simulink library "AeroSim"  (Simulink 7.8)
settings: Solver=ode45  StartTime=0.0  StopTime=10.0  RelTol=1e-3
libraries: AeroSim x3
settings Model: Creator=Ryan  LastModifiedBy=Ryan

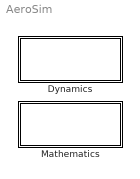
== system AeroSim ==
  Dynamics : Subsystem
      mask Display: disp('Dynamics')
  Mathematics : Subsystem
      mask Display: disp('Mathematics')

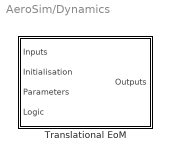
== system AeroSim/Dynamics ==
  Translational EoM : Subsystem

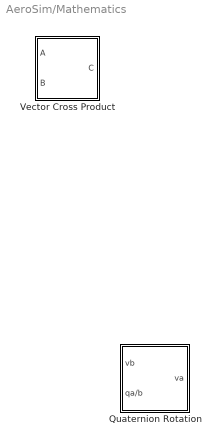
== system AeroSim/Mathematics ==
  Quaternion Rotation : Subsystem
  Vector Cross Product : Subsystem

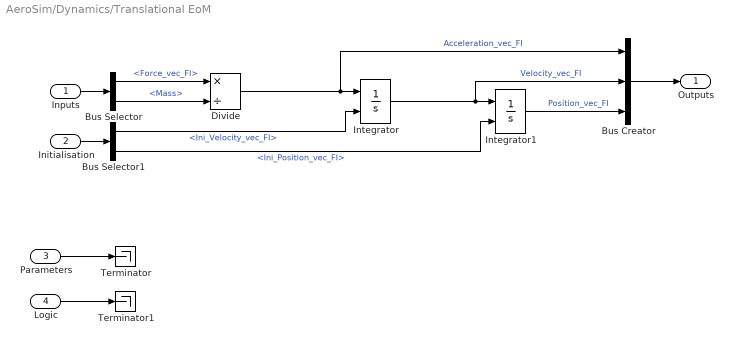
== system AeroSim/Dynamics/Translational EoM ==
  Inputs : Inport  OutDataTypeStr=Bus: Dynamics_TranslationalEoM_Inputs
  Initialisation : Inport  Port=2  OutDataTypeStr=Bus: Dynamics_TranslationalEoM_Initialisation
  Parameters : Inport  Port=3
  Logic : Inport  Port=4
  Bus Creator : BusCreator  Inputs=3
  Bus Selector : BusSelector  OutputSignals=Force_vec_FI,Mass
  Bus Selector1 : BusSelector  OutputSignals=Ini_Velocity_vec_FI,Ini_Position_vec_FI
  Divide : Product  Inputs=*/
  Integrator : Integrator  InitialConditionSource=external
  Integrator1 : Integrator  InitialConditionSource=external
  Terminator : Terminator
  Terminator1 : Terminator
  Outputs : Outport  OutDataTypeStr=Bus: Dynamics_TranslationalEoM_Outputs
  wires:
  Parameters/1 -> Terminator/1
  Logic/1 -> Terminator1/1
  Inputs/1 -> Bus Selector/1
  Bus Selector/1 -> Divide/1  "<Force_vec_FI>"
  Bus Selector/2 -> Divide/2  "<Mass>"
  Initialisation/1 -> Bus Selector1/1
  Bus Creator/1 -> Outputs/1
  Divide/1 -> Integrator/1, Bus Creator/1  "Acceleration_vec_FI"
  Bus Selector1/1 -> Integrator/2  "<Ini_Velocity_vec_FI>"
  Integrator/1 -> Integrator1/1, Bus Creator/2  "Velocity_vec_FI"
  Bus Selector1/2 -> Integrator1/2  "<Ini_Position_vec_FI>"
  Integrator1/1 -> Bus Creator/3  "Position_vec_FI"

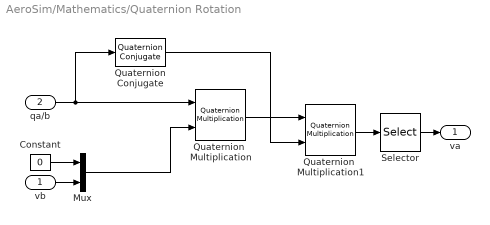
== system AeroSim/Mathematics/Quaternion Rotation ==
  vb : Inport
  qa/b : Inport  Port=2
  Constant : Constant  Value=0
  Mux : Mux  Inputs=2
  Quaternion Conjugate : AeroSim/Mathematics/Quaternion Conjugate
  Quaternion  Multiplication : AeroSim/Mathematics/Quaternion Multiplication
  Quaternion  Multiplication1 : AeroSim/Mathematics/Quaternion Multiplication
  Selector : Selector  InputPortWidth=4  IndexOptions=Index vector (dialog)  Indices=[2 3 4]  OutputSizes=1
  va : Outport
  wires:
  vb/1 -> Mux/2
  Constant/1 -> Mux/1
  qa/b/1 -> Quaternion  Multiplication/1, Quaternion Conjugate/1
  Mux/1 -> Quaternion  Multiplication/2
  Quaternion  Multiplication/1 -> Quaternion  Multiplication1/1
  Quaternion  Multiplication1/1 -> Selector/1
  Selector/1 -> va/1
  Quaternion Conjugate/1 -> Quaternion  Multiplication1/2

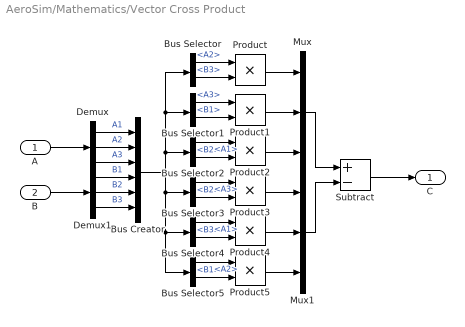
== system AeroSim/Mathematics/Vector Cross Product ==
  A : Inport
  B : Inport  Port=2
  Bus Creator : BusCreator  Inputs=6
  Bus Selector : BusSelector  OutputSignals=A2,B3
  Bus Selector1 : BusSelector  OutputSignals=A3,B1
  Bus Selector2 : BusSelector  OutputSignals=A1,B2
  Bus Selector3 : BusSelector  OutputSignals=A3,B2
  Bus Selector4 : BusSelector  OutputSignals=A1,B3
  Bus Selector5 : BusSelector  OutputSignals=A2,B1
  Demux : Demux  Outputs=3
  Demux1 : Demux  Outputs=3
  Mux : Mux  Inputs=3
  Mux1 : Mux  Inputs=3
  Product{,1..5} (6 alike) : Product  RndMeth=Zero
  Subtract : Sum  Inputs=+-
  C : Outport
  wires:
  Subtract/1 -> C/1
  Bus Creator/1 -> Bus Selector4/1, Bus Selector5/1, Bus Selector3/1, Bus Selector2/1, Bus Selector1/1, Bus Selector/1
  Mux1/1 -> Subtract/2
  Mux/1 -> Subtract/1
  Product5/1 -> Mux1/3
  Product4/1 -> Mux1/2
  Product3/1 -> Mux1/1
  Product2/1 -> Mux/3
  Product1/1 -> Mux/2
  Product/1 -> Mux/1
  Bus Selector5/2 -> Product5/2  "<B1>"
  Bus Selector5/1 -> Product5/1  "<A2>"
  Bus Selector4/2 -> Product4/2  "<B3>"
  Bus Selector4/1 -> Product4/1  "<A1>"
  Bus Selector3/2 -> Product3/2  "<B2>"
  Bus Selector3/1 -> Product3/1  "<A3>"
  Bus Selector2/2 -> Product2/2  "<B2>"
  Bus Selector2/1 -> Product2/1  "<A1>"
  Bus Selector1/2 -> Product1/2  "<B1>"
  Bus Selector1/1 -> Product1/1  "<A3>"
  Bus Selector/2 -> Product/2  "<B3>"
  Bus Selector/1 -> Product/1  "<A2>"
  Demux1/3 -> Bus Creator/6  "B3"
  Demux1/2 -> Bus Creator/5  "B2"
  Demux1/1 -> Bus Creator/4  "B1"
  Demux/3 -> Bus Creator/3  "A3"
  Demux/2 -> Bus Creator/2  "A2"
  Demux/1 -> Bus Creator/1  "A1"
  B/1 -> Demux1/1
  A/1 -> Demux/1
